simulink model "testpitch"  (R2025b)
settings: Solver=VariableStepAuto  StartTime=0.0  StopTime=20  RelTol=1e-3
undefined symbols (not defined in the file): CG, LongInertia, Mass, RotateInertia, Time
libraries: slpidlib x1
settings Model: Creator=Alienware R7  LastModifiedBy=Alienware R7

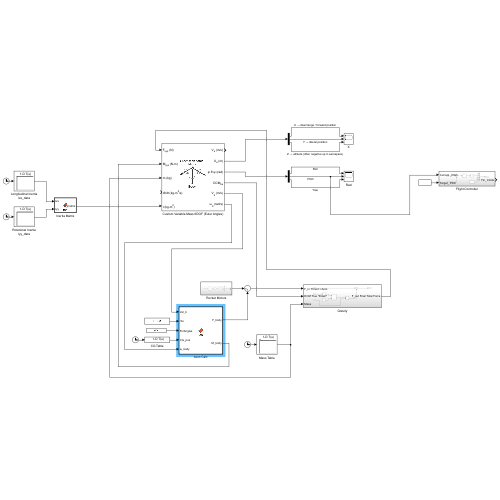
[thumbnail: Simulink's stored preview of the top-level diagram]
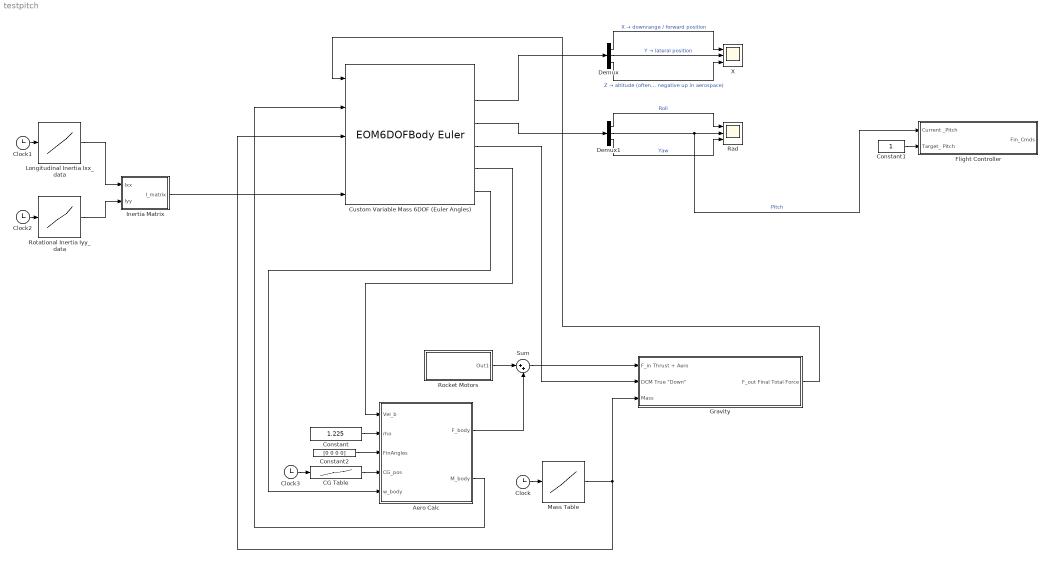
== system testpitch ==
  Aero Calc : MATLAB Function  TreatAsAtomicUnit=on
  CG Table : Lookup_n-D  NumberOfTableDimensions=1  BreakpointsForDimension1=Time  Table=CG  InternalRulePriority=Speed  RndMeth=Simplest
  Clock{,1..3} (4 alike) : Clock
  Constant : Constant  Value=1.225
  Constant1 : Constant
  Constant2 : Constant  Value=[0 0 0 0]
  Custom Variable Mass 6DOF (Euler Angles) : EOM6DOFBodyEuler  mtype=Custom Variable
  Demux : Demux  Outputs=3
  Demux1 : Demux  Outputs=3
  Flight Controller : Subsystem
  Gravity : Subsystem
  Inertia Matrix : MATLAB Function  TreatAsAtomicUnit=on
  Longitudinal Inertia Ixx_data : Lookup_n-D  NumberOfTableDimensions=1  BreakpointsForDimension1=Time  Table=LongInertia  InternalRulePriority=Speed  RndMeth=Simplest
  Mass Table : Lookup_n-D  NumberOfTableDimensions=1  BreakpointsForDimension1=Time  Table=Mass  InternalRulePriority=Speed  RndMeth=Simplest
  Rad : Scope  NumInputPorts=3
      settings: ActiveDisplayYMinimum=-5.637799594233627  ActiveDisplayYMaximum=5.49894876931758
  Rocket Motors : Subsystem
  Rotational Inertia Iyy_data : Lookup_n-D  NumberOfTableDimensions=1  BreakpointsForDimension1=Time  Table=RotateInertia  InternalRulePriority=Speed  RndMeth=Simplest
  Sum : Sum  Inputs=|++
  X : Scope  NumInputPorts=3
      settings: ActiveDisplayYMinimum=-232.47693637403665  ActiveDisplayYMaximum=666.30607714770417
  wires:
  Rocket Motors/1(Out1) -> Sum/1
  Longitudinal Inertia Ixx_data/1 -> Inertia Matrix/1(Ixx)
  Rotational Inertia Iyy_data/1 -> Inertia Matrix/2(Iyy)
  Custom Variable Mass 6DOF (Euler Angles)/5 -> Aero Calc/1(Vel_b)
  CG Table/1 -> Aero Calc/4(CG_pos)
  Constant/1 -> Aero Calc/2(rho)
  Aero Calc/2(M_body) -> Custom Variable Mass 6DOF (Euler Angles)/2
  Aero Calc/1(F_body) -> Sum/2
  Sum/1 -> Gravity/1(F_in Thrust + Aero)
  Custom Variable Mass 6DOF (Euler Angles)/4 -> Gravity/2("DCM True \"Down\"")
  Mass Table/1 -> Custom Variable Mass 6DOF (Euler Angles)/3, Gravity/3(Mass)
  Gravity/1(F_out Final Total Force) -> Custom Variable Mass 6DOF (Euler Angles)/1
  Clock/1 -> Mass Table/1
  Clock1/1 -> Longitudinal Inertia Ixx_data/1
  Clock2/1 -> Rotational Inertia Iyy_data/1
  Clock3/1 -> CG Table/1
  Inertia Matrix/1(I_matrix) -> Custom Variable Mass 6DOF (Euler Angles)/5
  Custom Variable Mass 6DOF (Euler Angles)/6 -> Aero Calc/5(w_body)
  Custom Variable Mass 6DOF (Euler Angles)/2 -> Demux/1
  Custom Variable Mass 6DOF (Euler Angles)/3 -> Demux1/1
  Demux1/1 -> Rad/1  "Roll"
  Demux1/2 -> Flight Controller/1(Current _Pitch), Rad/2  "Pitch"
  Demux/2 -> X/2  "Y → lateral position"
  Demux1/3 -> Rad/3  "Yaw"
  Demux/3 -> X/3  "Z → altitude (often negative up in aerospace)"
  Demux/1 -> X/1  "X → downrange / forward position"
  Constant1/1 -> Flight Controller/2(Target_ Pitch)
  Constant2/1 -> Aero Calc/3(FinAngles)

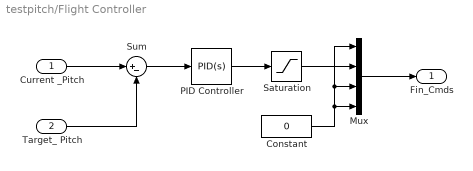
== system testpitch/Flight Controller ==
  Current _Pitch : Inport
  Target_ Pitch : Inport  Port=2
  Constant : Constant  Value=0
  Mux : Mux
  PID Controller : slpidlib/PID Controller  Controller=PID  Form=Parallel  TimeDomain=Continuous-time  UseExternalTs=off  SampleTime=-1  IntegratorMethod=Forward Euler  FilterMethod=Forward Euler  ControllerParametersSource=internal  P=-0.03  I=0  UseKiTs=off  D=-0.01  UseExternalDerivativeSource=off  N=100  UseFilter=on  TunerSelectOption=Transfer Function Based (PID Tuner App)  InitialConditionSource=internal  InitialConditionForIntegrator=0  InitialConditionForFilter=0  DifferentiatorICPrevScaledInput=0  ExternalReset=none  TrackingMode=off  Kt=1  LimitOutput=off  SatLimitsSource=internal  UpperSaturationLimit=inf  LowerSaturationLimit=-inf  LinearizeAsGain=on  AntiWindupMode=none  Kb=1  LimitIntegrator=off  UpperIntegratorSaturationLimit=inf  LowerIntegratorSaturationLimit=-inf  POutMin=[]  POutMax=[]  IOutMin=[]  IOutMax=[]  DOutMin=[]  DOutMax=[]  NOutMin=[]  NOutMax=[]  SumOutMin=[]  SumOutMax=[]  SaturationOutMin=[]  SaturationOutMax=[]  PParamMin=[]  PParamMax=[]  IParamMin=[]  IParamMax=[]  DParamMin=[]  DParamMax=[]  NParamMin=[]  NParamMax=[]  KbParamMin=[]  KbParamMax=[]  KtParamMin=[]  KtParamMax=[]  KbOutMin=[]  KbOutMax=[]  KtOutMin=[]  KtOutMax=[]  IntegratorOutMin=[]  IntegratorOutMax=[]  FilterOutMin=[]  FilterOutMax=[]  SumI1OutMin=[]  SumI1OutMax=[]  SumI2OutMin=[]  SumI2OutMax=[]  SumI3OutMin=[]  SumI3OutMax=[]  SumI4OutMin=[]  SumI4OutMax=[]  SumDOutMin=[]  SumDOutMax=[]  DifferentiatorOutMin=[]  DifferentiatorOutMax=[]  FilterDiffOutCoefMin=[]  FilterDiffOutCoefMax=[]  ReciprocalOutMin=[]  ReciprocalOutMax=[]  SumDenOutMin=[]  SumDenOutMax=[]  SumNumOutMin=[]  SumNumOutMax=[]  DivideOutMin=[]  DivideOutMax=[]  UdiffTsProdOutMin=[]  UdiffTsProdOutMax=[]  NTsProdOutMin=[]  NTsProdOutMax=[]  UintegralTsProdOutMin=[]  UintegralTsProdOutMax=[]  UngainTsProdOutMin=[]  UngainTsProdOutMax=[]  ClampingZeroOutDataTypeStr=Inherit: Inherit via back propagation  ClampingZeroOutMin=[]  ClampingZeroOutMax=[]  FilterDenConstantOutDataTypeStr=Inherit: Inherit via back propagation  FilterDenConstantOutMin=[]  FilterDenConstantOutMax=[]  PCopyOutDataTypeStr=Inherit: Inherit via back propagation  PCopyOutMin=[]  PCopyOutMax=[]  NCopyOutDataTypeStr=Inherit: Inherit via back propagation  NCopyOutMin=[]  NCopyOutMax=[]  IntegratorContinuousStateAttributes=''  IntegratorStateMustResolveToSignalObject=off  IntegratorRTWStateStorageClass=Auto  FilterContinuousStateAttributes=''  FilterStateMustResolveToSignalObject=off  FilterRTWStateStorageClass=Auto  ParallelPVariant=InternalParameters  IdealPVariant=Disabled  IVariant=InternalParameters  DVariant=InternalParameters  IntegratorVariant=Continuous  SatVariant=Disabled  AWVariant=Passthrough  PCopyVariant=Disabled  TRVariant=Disabled  FdbkBlocksVariant=Forward  IdealPFdbkVariant=Disabled  SatFdbkVariant=Disabled  DerivativeFilterVariant=ContFilter  NVariant=InternalParameters  NCopyVariant=Disabled  FilterICVariant=InternalICsFilter  IntegratorICVariant=InternalICs  ExternalResetVariant=Disabled  TRSumVariant=Passthrough  SumFdbkVariant=Disabled  SumVariant=Sum_PID  TsampFilterVariant=InternalTs  TsampNgainVariant=Passthrough  TsampIntegralVariant=Disabled_SignalSpec  ExternalSaturationOutDataTypeStr=Inherit: Same as second input  DerivativeSourceVariant=ErrorSignal  PreIntVariant=InternalPreInt
  Saturation : Saturate  UpperLimit=0.26  LowerLimit=-0.26
  Sum : Sum  Inputs=|+-
  Fin_Cmds : Outport
  wires:
  Target_ Pitch/1 -> Sum/2
  Current _Pitch/1 -> Sum/1
  Sum/1 -> PID Controller/1
  PID Controller/1 -> Saturation/1
  Saturation/1 -> Mux/2
  Constant/1 -> Mux/3, Mux/1, Mux/4
  Mux/1 -> Fin_Cmds/1

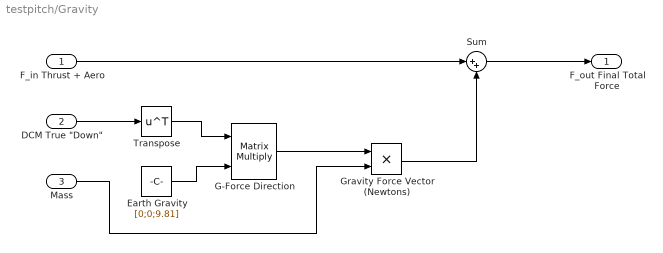
== system testpitch/Gravity ==
  F_in Thrust + Aero : Inport
  "DCM True \"Down\"" : Inport  Port=2
  Mass : Inport  Port=3
  Earth Gravity : Constant  Value=[0;0;9.81]
  G-Force Direction : Product  Multiplication=Matrix(*)
  Gravity Force Vector (Newtons) : Product
  Sum : Sum  Inputs=|++
  Transpose : Math  Operator=transpose
  F_out Final Total Force : Outport
  wires:
  "DCM True \"Down\""/1 -> Transpose/1
  Transpose/1 -> G-Force Direction/1
  Earth Gravity/1 -> G-Force Direction/2
  G-Force Direction/1 -> Gravity Force Vector (Newtons)/1
  Mass/1 -> Gravity Force Vector (Newtons)/2
  F_in Thrust + Aero/1 -> Sum/1
  Gravity Force Vector (Newtons)/1 -> Sum/2
  Sum/1 -> F_out Final Total Force/1

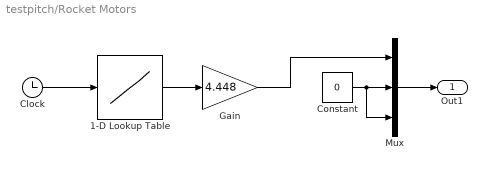
== system testpitch/Rocket Motors ==
  1-D Lookup Table : Lookup_n-D  NumberOfTableDimensions=1  BreakpointsForDimension1=[0;0.125;0.25;0.375;0.5;0.625;0.75;0.875;1;1.125;1.25;100]  Table=[0;31;36;41;41;46;55;60;58;50;0;0]  InternalRulePriority=Speed  RndMeth=Simplest
  Clock : Clock
  Constant : Constant  Value=0
  Gain : Gain  Gain=4.448
  Mux : Mux  Inputs=3
  Out1 : Outport
  wires:
  Clock/1 -> 1-D Lookup Table/1
  1-D Lookup Table/1 -> Gain/1
  Constant/1 -> Mux/2, Mux/3
  Gain/1 -> Mux/1
  Mux/1 -> Out1/1

== matlab function testpitch/Aero Calc ==
  data: Vel_b input; F_body output; rho input; FinAngles input; CG_pos input; M_body output; w_body input
function [F_body, M_body] = fcn(Vel_b, rho, FinAngles, CG_pos, w_body)
    % --- 1. SETUP & CONSTANTS ---
    % ---------------------------------------------------------
    % UNPACK INPUTS
    u = Vel_b(1); % Forward Velocity
    v = Vel_b(2); % Side Velocity (not used for pitch)
    w = Vel_b(3); % Down Velocity
    
    % CALCULATE TOTAL VELOCITY (Magnitude)
    V = sqrt(u^2 + w^2);
    
    % PREVENT DIVIDE BY ZERO AT LAUNCH
    if V < 0.1
        V = 0.1;
    end
    
    % --- YOUR ROCKET DATA ---
    % Rear Fins (4 Fins, Area 28.4 cm^2 each)
    S_rear_one    = 0.00284;  % Converted to m^2
    Num_fins_rear = 4;
    CL_alpha_rear = 3.0;      % Approx lift slope
    
    % Canards (4 Fins, Area 12.9 cm^2 each)
    S_canard_one    = 0.00129; % Converted to m^2
    Num_fins_canard = 4;
    CL_alpha_canard = 2.5;     
    
    % Reference Area (Cross section of body tube)
    A_ref = 0.00456; 
    
    % LOCATIONS (Distance from Nose Cone in Meters)
    X_canard_loc  = 0.18;      % Tip + 18cm
    
    Rocket_Length = 0.683;     % Total length of your rocket
    X_rear_loc    = Rocket_Length; % Fins are at the very bottom
    
    
    % --- 2. EXISTING AERODYNAMICS (STATIC) ---
    % ---------------------------------------------------------
    % CALCULATE ANGLE OF ATTACK (Alpha) WITH LOW SPEED PROTECTION
    % This fixes the violent spikes at apogee!
    if V < 1.0
        alpha = 0;           % Prevent glitches when stopped
    else
        alpha = atan2(w, u); % Calculate real angle
    end
    
    % CALCULATE DYNAMIC PRESSURE
    q_dynamic = 0.5 * rho * V^2;
    
    % CALCULATE LIFT FORCE (Main Body + Fins Static)
    % FinAngles(2) is the Pitch Command
    Total_Angle = alpha + FinAngles(2);
    
    % Note: Summing lift from fins approx:
    Cl_total = (Num_fins_rear * CL_alpha_rear * S_rear_one)/A_ref; 
    
    F_lift = q_dynamic * A_ref * Cl_total * Total_Angle;
    
    % CALCULATE DRAG FORCE (Simplified)
    Cd = 1.3;
    F_drag = q_dynamic * A_ref * Cd;
    
    % OUTPUT FORCES [Fx, Fy, Fz] -> [Drag, Side, Lift]
    % Drag acts back (-x), Lift acts up (-z in body frame)
    F_body = [-F_drag; 0; -F_lift];
    
    
    % --- 3. MOMENTS & DAMPING ---
    % ---------------------------------------------------------
    % A. STATIC MOMENT (The "Spring")
    % Your CP location (approximate center of lift of fins)
    CP_location = X_rear_loc; 
    
    % STABILITY FIX: Lever arm is (CG - CP) for restoring moment
    lever_arm_static = CG_pos(1) - CP_location;
    
    Moment_Pitch_Static = F_lift * lever_arm_static;
    
    
    % B. DAMPING MOMENT (The "Shock Absorber")
    % Pitch Rate (q) is the 2nd element of w_body
    q_rate = w_body(2); 
    
    % Calculate Damping Levers (Distance from CURRENT CG)
    L_arm_rear   = X_rear_loc - CG_pos(1);    % Positive (Behind CG)
    L_arm_canard = X_canard_loc - CG_pos(1);  % Negative (In Front of CG)

    % Calculate Damping Factor (Resistance force * Distance)
    % Using 2 fins effective for pitch plane out of 4
    Damp_Factor_Rear   = 0.5 * rho * V * (S_rear_one * 2)   * CL_alpha_rear   * L_arm_rear^2;
    Damp_Factor_Canard = 0.5 * rho * V * (S_canard_one * 2) * CL_alpha_canard * L_arm_canard^2;

    % Total Damping Moment (Opposes rotation)
    Moment_Damping = -(Damp_Factor_Rear + Damp_Factor_Canard) * q_rate;
    
    
    % --- 4. FINAL MOMENT OUTPUT ---
    % ---------------------------------------------------------
    Total_Pitch_Moment = Moment_Pitch_Static + Moment_Damping;
    
    % [Roll, Pitch, Yaw]
    M_body = [0; Total_Pitch_Moment; 0];
    
end

== matlab function testpitch/Inertia Matrix ==
  data: Ixx input; I_matrix output; Iyy input
function I_matrix = fcn(Ixx, Iyy)
    % Create a 3x3 Inertia Tensor
    % Rockets are symmetric, so we put Zeros in the corners.
    % Ixx is Roll Inertia. Iyy is Pitch/Yaw Inertia.
    
    I_matrix = [Ixx,  0,    0; 
                 0,  Iyy,   0; 
                 0,   0,   Iyy];
end
